simulink model "ES248B_MotAgArbn"  (R2013b)
settings: Solver=FixedStepDiscrete  SolverMode=SingleTasking  StartTime=0.0  StopTime=1  FixedStep=0.0005  RelTol=1e-3
values from neighbouring files (symbols this model uses):
  MAXSTALL_CNT_U08 = DataDict.Constant    [ES248B_MotAgArbn_DataDict.m]
undefined symbols (not defined in the file or in its folder): sigbuilder_block
libraries: simulink x4
settings Model: ModifiedHistory=Rev 008: Updated model to Matlab 2013B, added comments to show requirement linkage  Creator=nz3zln  LastModifiedBy=TZBSJD
settings SolverCC: AutoInsertRateTranBlk=on  InsertRTBMode=Always
settings DataIOCC: LimitDataPoints=off  SaveFormat=Structure  ReturnWorkspaceOutputs=on
settings OptimizationCC: BlockReduction=off  InlineParams=on  ZeroExternalMemoryAtStartup=off  ZeroInternalMemoryAtStartup=off  OptimizeModelRefInitCode=on  LifeSpan=1
settings DebuggingCC: SignalInfNanChecking=error  SignalRangeChecking=warning  UnderspecifiedInitializationDetection=Simplified  SolverPrmCheckMsg=error  InheritedTsInSrcMsg=error  DiscreteInheritContinuousMsg=error  SingleTaskRateTransMsg=error  TasksWithSamePriorityMsg=error  SigSpecEnsureSampleTimeMsg=error  CheckMatrixSingularityMsg=error  ParameterUnderflowMsg=error  ParameterPrecisionLossMsg=error  ParameterTunabilityLossMsg=error  FixptConstUnderflowMsg=warning  FixptConstOverflowMsg=warning  VectorMatrixConversionMsg=error  SignalLabelMismatchMsg=error  UnconnectedInputMsg=error  UnconnectedOutputMsg=error  UnconnectedLineMsg=error  SFcnCompatibilityMsg=error  UniqueDataStoreMsg=warning  BusObjectLabelMismatch=error  RootOutportRequireBusObject=error  AssertControl=DisableAll  ModelReferenceIOMsg=error  ModelReferenceVersionMismatchMessage=warning  ModelReferenceIOMismatchMessage=error  ModelReferenceCSMismatchMessage=warning  ModelReferenceDataLoggingMessage=error  StateNameClashWarn=warning  StrictBusMsg=ErrorOnBusTreatedAsVector  NonBusSignalsTreatedAsBus=error  SFUnexpectedBacktrackingDiag=error  SFInvalidInputDataAccessInChartInitDiag=error  SFNoUnconditionalDefaultTransitionDiag=error  SFTransitionOutsideNaturalParentDiag=error  SFUnconditionalTransitionShadowingDiag=error  SFUndirectedBroadcastEventsDiag=error
settings ModelReferenceCC: ModelReferenceNumInstancesAllowed=Single
settings RTWCC: SystemTargetFile=autosar.tlc  GenCodeOnly=on  TemplateMakefile=ert_default_tmf  Description=AUTOSAR  GenerateReport=on  ProcessScript=autosar_make_rtw_hook  LaunchReport=on
settings CodeAppCC: GenerateComments=off  IgnoreCustomStorageClasses=off  CustomSymbolStrType=$N$R$M  CustomSymbolStrBlkIO=$N$M  SimulinkBlockComments=off
settings STFCustomTargetCC: ParMdlRefBuildCompliant=on  CompOptLevelCompliant=on  IncludeMdlTerminateFcn=off  CombineOutputUpdateFcns=on  SuppressErrorStatus=on  ERTFirstTimeCompliant=on  ERTCustomFileBanners=on  SupportNonFinite=off  SupportComplex=off  SupportContinuousTime=off  SupportNonInlinedSFcns=off  MATLABClassNameForMDSCustomization=Simulink.SoftwareTarget.ERTCustomization  AutosarCompliant=on  GRTInterface=off  SystemTargetFile=autosar.tlc
settings ERTTargetCC: CodeReplacementLibrary=ANSI_C  ConcurrentExecutionCompliant=off  IncludeMdlTerminateFcn=off  SuppressErrorStatus=on  SupportNonFinite=off  SupportComplex=off  ModelStepFunctionPrototypeControlCompliant=off  CPPClassGenCompliant=off  AutosarCompliant=on  InlinedParameterPlacement=NonHierarchical  ERTCustomFileTemplate=example_file_process.tlc  EnableUserReplacementTypes=on

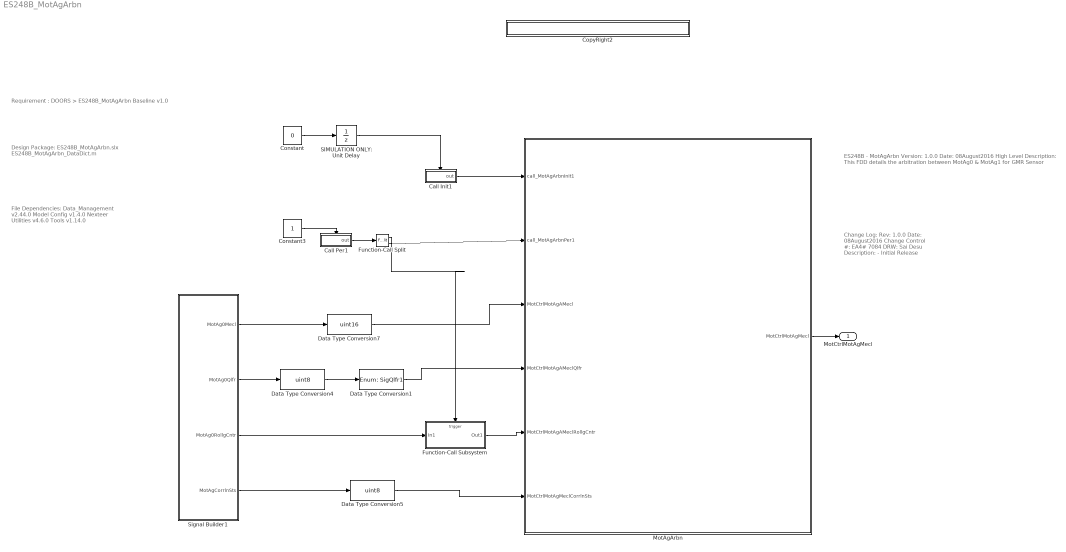
== system ES248B_MotAgArbn ==
  note: ES248B - MotAgArbn
      |
      | Version: 1.0.0
      | Date: 08August2016
      |
      | High Level Description:
      | This FDD details the arbitration between MotAg0 & MotAg1 for GMR Sensor
  note: Change Log:
      |
      | Rev: 1.0.0
      | Date: 08August2016
      | Change Control #: EA4# 7084
      | DRW: Sai Desu
      | Description:
      | - Initial Release
  note: File Dependencies:
      | Data_Management v2.44.0
      | Model Config v1.4.0
      | Nexteer Utilities v4.6.0
      | Tools v1.14.0
  note: Requirement :
      |
      | DOORS > ES248B_MotAgArbn  Baseline  v1.0
  note: Design Package:
      | ES248B_MotAgArbn.slx
      | ES248B_MotAgArbn_DataDict.m
  Call Init1 : Subsystem  TreatAsAtomicUnit=on
  Call Per1 : Subsystem  TreatAsAtomicUnit=on
  Constant : Constant  Value=0  OutDataTypeStr=uint8
  Constant3 : Constant  OutDataTypeStr=int8
  CopyRight2 : Subsystem  Description=|  mask(Copyright Information){none=on}
      | Copyright info block.                                               
      |                                                                     
      | Place copyright information at the top of every subsystem in design.
      mask prompts: none "No parameters"
      mask help: Place copyright information at the top of every subsystem in design.
      mask Display:
      | NxtrConf = 'Nexteer Confidential';
      | 
      | sys = bdroot; %handle for the current model ("system")
      | first = get_param(sys,'Created');
      | first = first(end-3:end);  %year is last four digits
      | 
      | last = get_param(sys,'LastModifiedDate');
      | if isempty(last)
      |     last = datestr(now,'yyyy');
      | else
      |     last = last(end-3:end);
      | end
      | 
      | if strcmp(first,last)
      |     fprintf('%s -- Copyright %s Nexteer',NxtrConf,first)
      | else
      |     fprintf('%s -- %s%s- %s Nexteer',NxtrConf,char(169),first,last)
      | end
  Data Type Conversion1 : DataTypeConversion  OutDataTypeStr=Enum: SigQlfr1
  Data Type Conversion4 : DataTypeConversion  OutDataTypeStr=uint8  RndMeth=Nearest
  Data Type Conversion5 : DataTypeConversion  OutDataTypeStr=uint8  RndMeth=Nearest
  Data Type Conversion7 : DataTypeConversion  OutDataTypeStr=uint16  RndMeth=Nearest
  Function-Call Split : FunctionCallSplit
  Function-Call Subsystem : Subsystem  TreatAsAtomicUnit=on
  MotAgArbn : Subsystem
  SIMULATION ONLY: Unit Delay : UnitDelay  InitialCondition=1  SampleTime=-1
  Signal Builder1 : Subsystem  Tag=STV Subsys  LoadFcn=sigbuilder_block('load');  StartFcn=sigbuilder_block('start');  StopFcn=sigbuilder_block('stop');  ClipboardFcn=sigbuilder_block('clipboard');  mask(Sigbuilder block){}
      mask help: Simulink:masks:SigbuilderBlock_MD
      mask init:
      | if ~strcmp(get_param(bdroot(gcbh),'SimulationStatus'),'stopped') tuvar = sigbuilder_block('maskInit'); end
      settings: CopyFcn=sigbuilder_block('copy');  DeleteFcn=sigbuilder_block('delete');  ModelCloseFcn=sigbuilder_block('modelClose');  PreSaveFcn=sigbuilder_block('preSave');  PauseFcn=sigbuilder_block('pause');  ContinueFcn=sigbuilder_block('continue');  NameChangeFcn=sigbuilder_block('namechange');  OpenFcn=sigbuilder_block('open',[1440 0 1440 753 ]);  CloseFcn=sigbuilder_block('close');
      mask Display: plot(0, 0, 100, 100,[2, 2, 32, 32, 2], [68, 8, 8, 68, 68],[32, 2], [38, 38], [32, 19, 2],[53, 60, 44], [32, 17, 17, 2],[16, 16, 31, 31]);txt = getActiveGroup(gcbh);text(2, 100, txt,'verticalAlignment', 'top');
  MotCtrlMotAgMecl : Outport
  wires:
  Constant3/1 -> Call Per1/Enable
  Call Per1/1(out) -> Function-Call Split/1
  Signal Builder1/4(MotAgCorrlnSts) -> Data Type Conversion5/1
  Signal Builder1/2(MotAg0Qlfr) -> Data Type Conversion4/1
  Signal Builder1/1(MotAg0Mecl) -> Data Type Conversion7/1
  Data Type Conversion4/1 -> Data Type Conversion1/1
  Data Type Conversion5/1 -> MotAgArbn/6(MotCtrlMotAgMeclCorrlnSts)
  Data Type Conversion7/1 -> MotAgArbn/3(MotCtrlMotAgAMecl)
  Function-Call Subsystem/1(Out1) -> MotAgArbn/5(MotCtrlMotAgAMeclRollgCntr)
  Signal Builder1/3(MotAg0RollgCntr) -> Function-Call Subsystem/1(In1)
  Function-Call Split/2 -> MotAgArbn/2(call_MotAgArbnPer1)
  Function-Call Split/1 -> Function-Call Subsystem/Trigger
  Call Init1/1(out) -> MotAgArbn/1(call_MotAgArbnInit1)
  Constant/1 -> SIMULATION ONLY: Unit Delay/1
  SIMULATION ONLY: Unit Delay/1 -> Call Init1/Enable
  MotAgArbn/1(MotCtrlMotAgMecl) -> MotCtrlMotAgMecl/1
  Data Type Conversion1/1 -> MotAgArbn/4(MotCtrlMotAgAMeclQlfr)

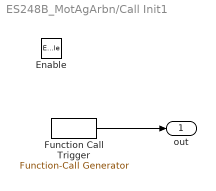
== system ES248B_MotAgArbn/Call Init1 ==
  Enable : EnablePort
  Function Call Trigger : simulink/Ports & Subsystems/Function-Call Generator  RequirementInfo={} %GIDa_03d3be70_2a53_4f3d_90ce_b287f92bdd04  sample_time=0.0005  numberOfIterations=1
  out : Outport
  wires:
  Function Call Trigger/1 -> out/1

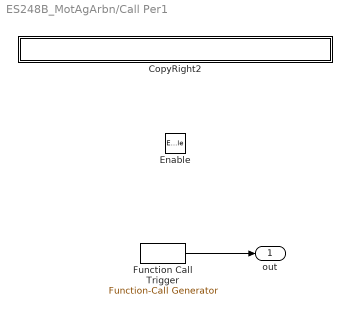
== system ES248B_MotAgArbn/Call Per1 ==
  Enable : EnablePort
  CopyRight2 : Subsystem  Description=|  mask(Copyright Information){none=on}
      | Copyright info block.                                               
      |                                                                     
      | Place copyright information at the top of every subsystem in design.
      mask prompts: none "No parameters"
      mask help: Place copyright information at the top of every subsystem in design.
      mask Display:
      | NxtrConf = 'Nexteer Confidential';
      | 
      | sys = bdroot; %handle for the current model ("system")
      | first = get_param(sys,'Created');
      | first = first(end-3:end);  %year is last four digits
      | 
      | last = get_param(sys,'LastModifiedDate');
      | if isempty(last)
      |     last = datestr(now,'yyyy');
      | else
      |     last = last(end-3:end);
      | end
      | 
      | if strcmp(first,last)
      |     fprintf('%s -- Copyright %s Nexteer',NxtrConf,first)
      | else
      |     fprintf('%s -- %s%s- %s Nexteer',NxtrConf,char(169),first,last)
      | end
  Function Call Trigger : simulink/Ports & Subsystems/Function-Call Generator  RequirementInfo={} %GIDa_6dd05ab1_f91b_4d7a_a0ec_1170d213fa7b  sample_time=0.0005  numberOfIterations=1
  out : Outport
  wires:
  Function Call Trigger/1 -> out/1

== system ES248B_MotAgArbn/CopyRight2 ==

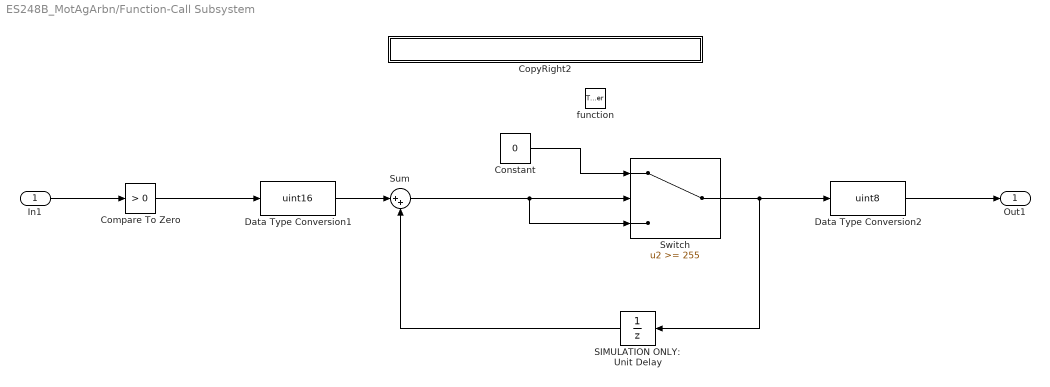
== system ES248B_MotAgArbn/Function-Call Subsystem ==
  In1 : Inport
  function : TriggerPort  TriggerType=function-call
  Compare To Zero : simulink/Logic and Bit Operations/Compare To Zero  relop=>  OutDataTypeStr=uint8
  Constant : Constant  Value=0  OutDataTypeStr=uint16
  CopyRight2 : Subsystem  Description=|  mask(Copyright Information){none=on}
      | Copyright info block.                                               
      |                                                                     
      | Place copyright information at the top of every subsystem in design.
      mask prompts: none "No parameters"
      mask help: Place copyright information at the top of every subsystem in design.
      mask Display:
      | NxtrConf = 'Nexteer Confidential';
      | 
      | sys = bdroot; %handle for the current model ("system")
      | first = get_param(sys,'Created');
      | first = first(end-3:end);  %year is last four digits
      | 
      | last = get_param(sys,'LastModifiedDate');
      | if isempty(last)
      |     last = datestr(now,'yyyy');
      | else
      |     last = last(end-3:end);
      | end
      | 
      | if strcmp(first,last)
      |     fprintf('%s -- Copyright %s Nexteer',NxtrConf,first)
      | else
      |     fprintf('%s -- %s%s- %s Nexteer',NxtrConf,char(169),first,last)
      | end
  Data Type Conversion1 : DataTypeConversion  OutDataTypeStr=uint16  RndMeth=Nearest
  Data Type Conversion2 : DataTypeConversion  OutDataTypeStr=uint8  RndMeth=Nearest
  SIMULATION ONLY: Unit Delay : UnitDelay  SampleTime=-1
  Sum : Sum  Inputs=|++
  Switch : Switch  Threshold=255
  Out1 : Outport
  wires:
  Constant/1 -> Switch/1
  Sum/1 -> Switch/3, Switch/2
  Data Type Conversion1/1 -> Sum/1
  Switch/1 -> SIMULATION ONLY: Unit Delay/1, Data Type Conversion2/1
  Data Type Conversion2/1 -> Out1/1
  SIMULATION ONLY: Unit Delay/1 -> Sum/2
  In1/1 -> Compare To Zero/1
  Compare To Zero/1 -> Data Type Conversion1/1

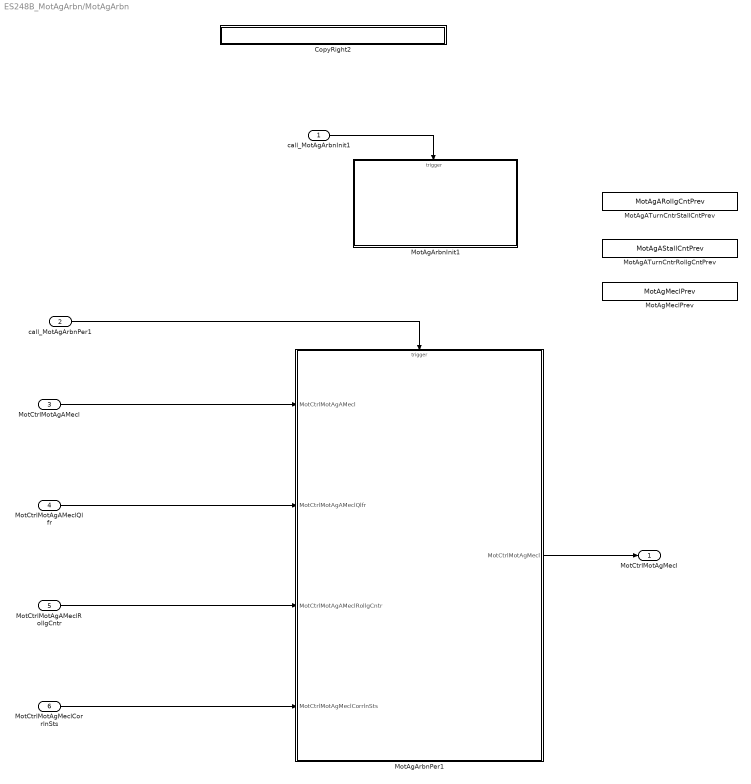
== system ES248B_MotAgArbn/MotAgArbn ==
  call_MotAgArbnInit1 : Inport  RequirementInfo={} %GIDa_2de43c09_82b6_47b9_8e99_1c21e4b82fe2
  call_MotAgArbnPer1 : Inport  RequirementInfo={} %GIDa_468d2479_6710_42ce_bd19_b69834ab6306  Port=2
  MotCtrlMotAgAMecl : Inport  Port=3
  MotCtrlMotAgAMeclQlfr : Inport  Port=4
  MotCtrlMotAgAMeclRollgCntr : Inport  RequirementInfo={} %GIDa_84fb02b3_72b4_4e28_a17f_e99f7297de00  Port=5
  MotCtrlMotAgMeclCorrlnSts : Inport  Port=6
  CopyRight2 : Subsystem  Description=|  mask(Copyright Information){none=on}
      | Copyright info block.                                               
      |                                                                     
      | Place copyright information at the top of every subsystem in design.
      mask prompts: none "No parameters"
      mask help: Place copyright information at the top of every subsystem in design.
      mask Display:
      | NxtrConf = 'Nexteer Confidential';
      | 
      | sys = bdroot; %handle for the current model ("system")
      | first = get_param(sys,'Created');
      | first = first(end-3:end);  %year is last four digits
      | 
      | last = get_param(sys,'LastModifiedDate');
      | if isempty(last)
      |     last = datestr(now,'yyyy');
      | else
      |     last = last(end-3:end);
      | end
      | 
      | if strcmp(first,last)
      |     fprintf('%s -- Copyright %s Nexteer',NxtrConf,first)
      | else
      |     fprintf('%s -- %s%s- %s Nexteer',NxtrConf,char(169),first,last)
      | end
  MotAgATurnCntrRollgCntPrev : DataStoreMemory  DataStoreName=MotAgAStallCntPrev  StateMustResolveToSignalObject=on
  MotAgATurnCntrStallCntPrev : DataStoreMemory  DataStoreName=MotAgARollgCntPrev  StateMustResolveToSignalObject=on
  MotAgArbnInit1 : Subsystem
  MotAgArbnPer1 : Subsystem  TreatAsAtomicUnit=on
  MotAgMeclPrev : DataStoreMemory  DataStoreName=MotAgMeclPrev  StateMustResolveToSignalObject=on
  MotCtrlMotAgMecl : Outport
  wires:
  call_MotAgArbnPer1/1 -> MotAgArbnPer1/Trigger
  MotAgArbnPer1/1(MotCtrlMotAgMecl) -> MotCtrlMotAgMecl/1
  MotCtrlMotAgAMecl/1 -> MotAgArbnPer1/1(MotCtrlMotAgAMecl)
  MotCtrlMotAgAMeclQlfr/1 -> MotAgArbnPer1/2(MotCtrlMotAgAMeclQlfr)
  MotCtrlMotAgMeclCorrlnSts/1 -> MotAgArbnPer1/4(MotCtrlMotAgMeclCorrlnSts)
  call_MotAgArbnInit1/1 -> MotAgArbnInit1/Trigger
  MotCtrlMotAgAMeclRollgCntr/1 -> MotAgArbnPer1/3(MotCtrlMotAgAMeclRollgCntr)

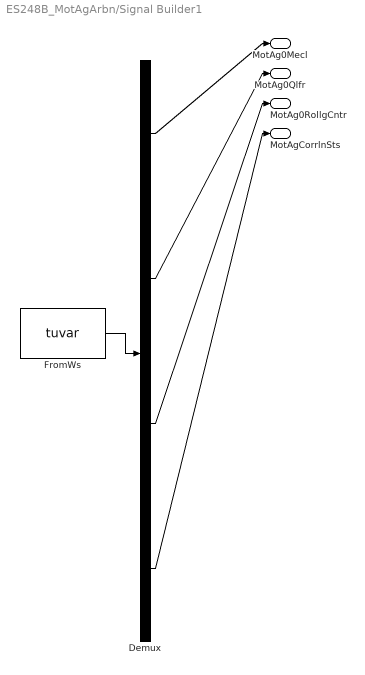
== system ES248B_MotAgArbn/Signal Builder1 ==
  Demux : Demux  Tag=STV Demux
  FromWs : FromWorkspace  Tag=STV FromWs  VariableName=tuvar  SampleTime=0
      SigBuilderData=|
      | common.afterFinalStr = 'Extrapolate'
      | common.sampleTime = 0
      | dataSet(1).timeRange = [0 1]
      | dataSet(1).name = 'Group 1'
      | dataSet(2).timeRange = [0 1]
      | dataSet(2).name = 'looping'
      | dataSet(3).timeRange = [0 1]
      | dataSet(3).name = 'TotalFial'
      | dataSet(4).timeRange = [0 1]
      | dataSet(4).name = 'Allpass'
      | sbobj.Groups(1).Name = 'Group 1'
      | sbobj.Groups(1).Signals(1).Name = 'MotAg0Mecl'
      | sbobj.Groups(1).Signals(1).XData = [0 0.166666666667 0.166666666667 0.333333333333 0.333333333333 0.5 0.5 0.666666666667 0.666666666667 0.833333333333 0.833333333333 0.901 0.901 1]
      | sbobj.Groups(1).Signals(1).YData = [0 65534 0 65534 0 65534 0 65534 0 65534 0 61000 0 60000]
      | sbobj.Groups(1).Signals(2).Name = 'MotAg0Qlfr'
      | sbobj.Groups(1).Signals(2).XData = [0 0.25 0.25 0.4 0.4 0.71 0.71 0.89 0.89 1]
      | sbobj.Groups(1).Signals(2).YData = [1 1 2 2 1 1 2 2 1 1]
      | sbobj.Groups(1).Signals(3).Name = 'MotAg0RollgCntr'
      | sbobj.Groups(1).Signals(3).XData = [0 1]
      | sbobj.Groups(1).Signals(3).YData = [1 1]
      | sbobj.Groups(1).Signals(4).Name = 'MotAgCorrlnSts'
      | sbobj.Groups(1).Signals(4).XData = [0 0.501 0.501 0.599 0.599 0.98 0.98 1]
      | sbobj.Groups(1).Signals(4).YData = [3 3 2 2 3 3 0 2]
      | sbobj.Groups(1).TimeRange = [0 1]
      | sbobj.Groups(2).Name = 'looping'
      | sbobj.Groups(2).Signals(1).Name = 'MotAg0Mecl'
      | sbobj.Groups(2).Signals(1).XData = [0 0.166666666667 0.166666666667 0.333333333333 0.333333333333 0.5 0.5 0.666666666667 0.666666666667 0.833333333333 0.833333333333 0.901 0.901 1]
      | sbobj.Groups(2).Signals(1).YData = [0 65534 0 65534 0 65534 0 65534 0 65534 0 61000 0 60000]
      | sbobj.Groups(2).Signals(2).Name = 'MotAg0Qlfr'
      | sbobj.Groups(2).Signals(2).XData = [0 0.25 0.4 0.71 0.71 0.89 0.89 1]
      | sbobj.Groups(2).Signals(2).YData = [1 1 1 1 2 2 1 1]
      | sbobj.Groups(2).Signals(3).Name = 'MotAg0RollgCntr'
      | sbobj.Groups(2).Signals(3).XData = [0 0.6 0.6 1]
      | sbobj.Groups(2).Signals(3).YData = [0 0 1 1]
      | sbobj.Groups(2).Signals(4).Name = 'MotAgCorrlnSts'
      | sbobj.Groups(2).Signals(4).XData = [0 0.201 0.201 0.3 0.3 0.501 0.599 0.633 0.633 0.667 0.667 0.98 0.98 1]
      | sbobj.Groups(2).Signals(4).YData = [3 3 1 1 3 3 3 3 0 0 3 3 0 2]
      | sbobj.Groups(2).TimeRange = [0 1]
      | sbobj.Groups(3).Name = 'TotalFial'
      | sbobj.Groups(3).Signals(1).Name = 'MotAg0Mecl'
      | sbobj.Groups(3).Signals(1).XData = [0 0.166666666667 0.166666666667 0.333333333333 0.333333333333 0.5 0.5 0.666666666667 0.666666666667 0.833333333333 0.833333333333 0.901 0.901 1]
      | sbobj.Groups(3).Signals(1).YData = [0 65534 0 65534 0 65534 0 65534 0 65534 0 61000 0 60000]
      | sbobj.Groups(3).Signals(2).Name = 'MotAg0Qlfr'
      | sbobj.Groups(3).Signals(2).XData = [0 0.04 0.04 0.1 0.25 0.4 0.7 0.7 0.89 0.89 1]
      | sbobj.Groups(3).Signals(2).YData = [2 2 1 1 1 1 1 2 2 1 1]
      | sbobj.Groups(3).Signals(3).Name = 'MotAg0RollgCntr'
      | sbobj.Groups(3).Signals(3).XData = [0 0.04 0.04 0.6 0.6 0.85 0.85 1]
      | sbobj.Groups(3).Signals(3).YData = [1 1 0 0 1 1 0 0]
      | sbobj.Groups(3).Signals(4).Name = 'MotAgCorrlnSts'
      | sbobj.Groups(3).Signals(4).XData = [0 0.201 0.201 0.3 0.3 0.501 0.599 0.599 0.7 0.7 0.98 0.98 1]
      | sbobj.Groups(3).Signals(4).YData = [3 3 1 1 3 3 3 0 0 3 3 0 2]
      | sbobj.Groups(3).TimeRange = [0 1]
      | sbobj.Groups(4).Name = 'Allpass'
      | sbobj.Groups(4).Signals(1).Name = 'MotAg0Mecl'
      | sbobj.Groups(4).Signals(1).XData = [0 0.166666666667 0.166666666667 0.333333333333 0.333333333333 0.5 0.5 0.666666666667 0.666666666667 0.833333333333 0.833333333333 0.901 0.901 1]
      | sbobj.Groups(4).Signals(1).YData = [0 65534 0 65534 0 65534 0 65534 0 65534 0 61000 0 60000]
      | sbobj.Groups(4).Signals(2).Name = 'MotAg0Qlfr'
      | sbobj.Groups(4).Signals(2).XData = [0 0.25 0.4 0.7 0.89 1]
      | sbobj.Groups(4).Signals(2).YData = [1 1 1 1 1 1]
      | sbobj.Groups(4).Signals(3).Name = 'MotAg0RollgCntr'
      | sbobj.Groups(4).Signals(3).XData = [0 0.6 0.89 1]
      | sbobj.Groups(4).Signals(3).YData = [1 1 1 1]
      | sbobj.Groups(4).Signals(4).Name = 'MotAgCorrlnSts'
      | sbobj.Groups(4).Signals(4).XData = [0 0.201 0.201 0.3 0.3 0.501 0.599 0.599 0.7 0.7 0.98 0.98 1]
      | sbobj.Groups(4).Signals(4).YData = [3 3 1 1 3 3 3 1 1 3 3 1 1]
      | sbobj.Groups(4).TimeRange = [0 1]
  MotAg0Mecl : Outport  Tag=STV Outport
  MotAg0Qlfr : Outport  Tag=STV Outport  Port=2
  MotAg0RollgCntr : Outport  Tag=STV Outport  Port=3
  MotAgCorrlnSts : Outport  Tag=STV Outport  Port=4
  wires:
  FromWs/1 -> Demux/1
  Demux/1 -> MotAg0Mecl/1
  Demux/2 -> MotAg0Qlfr/1
  Demux/3 -> MotAg0RollgCntr/1
  Demux/4 -> MotAgCorrlnSts/1

== system ES248B_MotAgArbn/Call Per1/CopyRight2 ==

== system ES248B_MotAgArbn/Function-Call Subsystem/CopyRight2 ==

== system ES248B_MotAgArbn/MotAgArbn/CopyRight2 ==

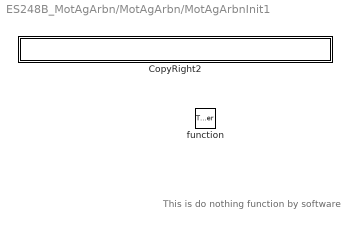
== system ES248B_MotAgArbn/MotAgArbn/MotAgArbnInit1 ==
  note: This is do nothing function by software
  function : TriggerPort  TriggerType=function-call
  CopyRight2 : Subsystem  Description=|  mask(Copyright Information){none=on}
      | Copyright info block.                                               
      |                                                                     
      | Place copyright information at the top of every subsystem in design.
      mask prompts: none "No parameters"
      mask help: Place copyright information at the top of every subsystem in design.
      mask Display:
      | NxtrConf = 'Nexteer Confidential';
      | 
      | sys = bdroot; %handle for the current model ("system")
      | first = get_param(sys,'Created');
      | first = first(end-3:end);  %year is last four digits
      | 
      | last = get_param(sys,'LastModifiedDate');
      | if isempty(last)
      |     last = datestr(now,'yyyy');
      | else
      |     last = last(end-3:end);
      | end
      | 
      | if strcmp(first,last)
      |     fprintf('%s -- Copyright %s Nexteer',NxtrConf,first)
      | else
      |     fprintf('%s -- %s%s- %s Nexteer',NxtrConf,char(169),first,last)
      | end

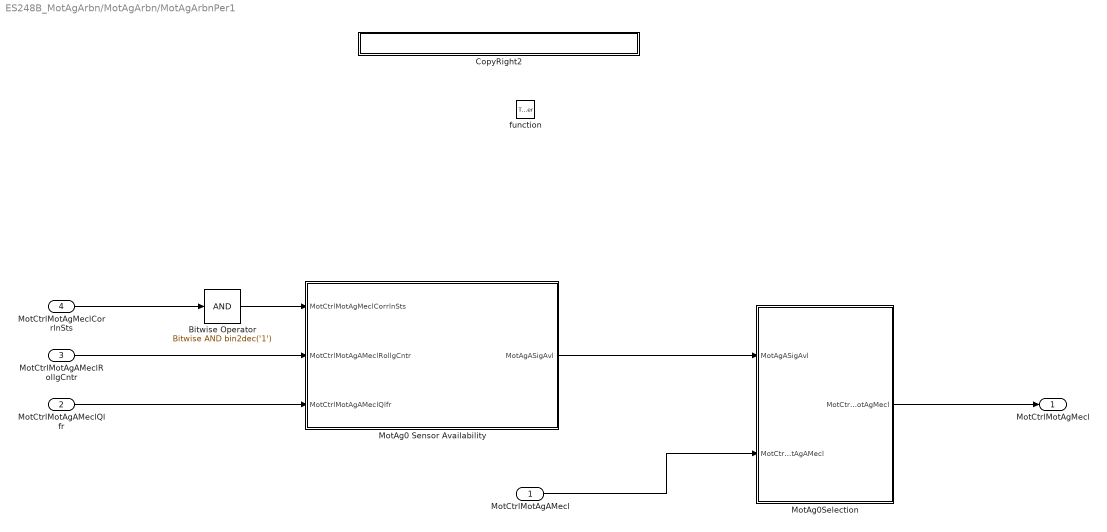
== system ES248B_MotAgArbn/MotAgArbn/MotAgArbnPer1 ==
  MotCtrlMotAgAMecl : Inport
  MotCtrlMotAgAMeclQlfr : Inport  Port=2
  MotCtrlMotAgAMeclRollgCntr : Inport  RequirementInfo={} %GIDa_9d4de4cc_7719_48bf_85c0_912168cfd52f  Port=3
  MotCtrlMotAgMeclCorrlnSts : Inport  Port=4
  function : TriggerPort  TriggerType=function-call
  Bitwise Operator : simulink/Logic and Bit Operations/Bitwise Operator  logicop=AND  UseBitMask=on  BitMask=bin2dec('1')  BitMaskRealWorld=Stored Integer
  CopyRight2 : Subsystem  Description=|  mask(Copyright Information){none=on}
      | Copyright info block.                                               
      |                                                                     
      | Place copyright information at the top of every subsystem in design.
      mask prompts: none "No parameters"
      mask help: Place copyright information at the top of every subsystem in design.
      mask Display:
      | NxtrConf = 'Nexteer Confidential';
      | 
      | sys = bdroot; %handle for the current model ("system")
      | first = get_param(sys,'Created');
      | first = first(end-3:end);  %year is last four digits
      | 
      | last = get_param(sys,'LastModifiedDate');
      | if isempty(last)
      |     last = datestr(now,'yyyy');
      | else
      |     last = last(end-3:end);
      | end
      | 
      | if strcmp(first,last)
      |     fprintf('%s -- Copyright %s Nexteer',NxtrConf,first)
      | else
      |     fprintf('%s -- %s%s- %s Nexteer',NxtrConf,char(169),first,last)
      | end
  MotAg0 Sensor Availability : Subsystem  RequirementInfo={} %GIDa_a3666822_1018_404e_9f7a_19faaace6442  TreatAsAtomicUnit=on
  MotAg0Selection : Subsystem  RequirementInfo={} %GIDa_85a2964f_79da_4020_bfb6_043b97388858
  MotCtrlMotAgMecl : Outport
  wires:
  MotCtrlMotAgMeclCorrlnSts/1 -> Bitwise Operator/1
  Bitwise Operator/1 -> MotAg0 Sensor Availability/1(MotCtrlMotAgMeclCorrlnSts)
  MotCtrlMotAgAMeclQlfr/1 -> MotAg0 Sensor Availability/3(MotCtrlMotAgAMeclQlfr)
  MotAg0 Sensor Availability/1(MotAgASigAvl) -> MotAg0Selection/1(MotAgASigAvl)
  MotCtrlMotAgAMecl/1 -> MotAg0Selection/2(MotCtrlMotAgAMecl)
  MotCtrlMotAgAMeclRollgCntr/1 -> MotAg0 Sensor Availability/2(MotCtrlMotAgAMeclRollgCntr)
  MotAg0Selection/1("MotCtrlMotAgMecl ") -> MotCtrlMotAgMecl/1

== system ES248B_MotAgArbn/MotAgArbn/MotAgArbnInit1/CopyRight2 ==

== system ES248B_MotAgArbn/MotAgArbn/MotAgArbnPer1/CopyRight2 ==

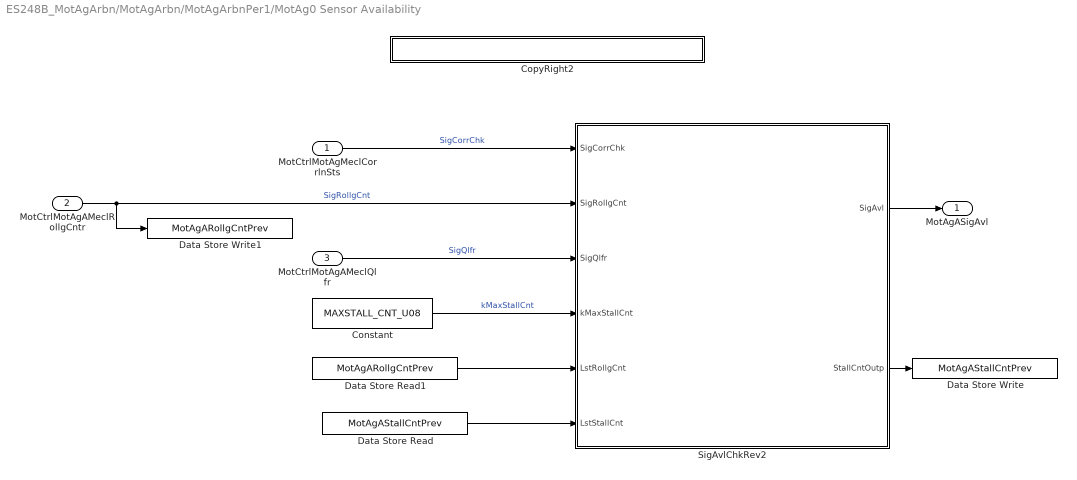
== system ES248B_MotAgArbn/MotAgArbn/MotAgArbnPer1/MotAg0 Sensor Availability ==
  MotCtrlMotAgMeclCorrlnSts : Inport
  MotCtrlMotAgAMeclRollgCntr : Inport  Port=2
  MotCtrlMotAgAMeclQlfr : Inport  Port=3
  Constant : Constant  Value=MAXSTALL_CNT_U08
  CopyRight2 : Subsystem  Description=|  mask(Copyright Information){none=on}
      | Copyright info block.                                               
      |                                                                     
      | Place copyright information at the top of every subsystem in design.
      mask prompts: none "No parameters"
      mask help: Place copyright information at the top of every subsystem in design.
      mask Display:
      | NxtrConf = 'Nexteer Confidential';
      | 
      | sys = bdroot; %handle for the current model ("system")
      | first = get_param(sys,'Created');
      | first = first(end-3:end);  %year is last four digits
      | 
      | last = get_param(sys,'LastModifiedDate');
      | if isempty(last)
      |     last = datestr(now,'yyyy');
      | else
      |     last = last(end-3:end);
      | end
      | 
      | if strcmp(first,last)
      |     fprintf('%s -- Copyright %s Nexteer',NxtrConf,first)
      | else
      |     fprintf('%s -- %s%s- %s Nexteer',NxtrConf,char(169),first,last)
      | end
  Data Store Read : DataStoreRead  DataStoreName=MotAgAStallCntPrev
  Data Store Read1 : DataStoreRead  DataStoreName=MotAgARollgCntPrev
  Data Store Write : DataStoreWrite  RequirementInfo={} %GIDa_9a9cd5ba_32cc_4b15_9fbb_ffc99f86186c  DataStoreName=MotAgAStallCntPrev
  Data Store Write1 : DataStoreWrite  RequirementInfo={} %GIDa_68fbb913_cad7_4656_a0fb_1b4163fceb61  DataStoreName=MotAgARollgCntPrev
  SigAvlChkRev2 : Stateflow chart  RequirementInfo="{'linktype_rmi_doors' '00011b4a (/ESG Group/FDD Module Requirements/EA4 Specific/ES248B_MotAgArbn)' '#ES248B_35' 'true' 'REQ:  ES248B_35' '' } %GIDa_ec1912f1_c7f6_4114_866c_684914a13f21"  TreatAsAtomicUnit=on
  MotAgASigAvl : Outport  RequirementInfo="{'linktype_rmi_doors' '00011b4a (/ESG Group/FDD Module Requirements/EA4 Specific/ES248B_MotAgArbn)' '#ES248B_35' 'true' 'REQ:  ES248B_35' '' } %GIDa_8d8daaab_601a_421a_88d3_d4e0374f5eae"
  wires:
  MotCtrlMotAgMeclCorrlnSts/1 -> SigAvlChkRev2/1(SigCorrChk)  "SigCorrChk"
  MotCtrlMotAgAMeclRollgCntr/1 -> Data Store Write1/1, SigAvlChkRev2/2(SigRollgCnt)  "SigRollgCnt"
  MotCtrlMotAgAMeclQlfr/1 -> SigAvlChkRev2/3(SigQlfr)  "SigQlfr"
  Constant/1 -> SigAvlChkRev2/4(kMaxStallCnt)  "kMaxStallCnt"
  SigAvlChkRev2/1(SigAvl) -> MotAgASigAvl/1
  Data Store Read1/1 -> SigAvlChkRev2/5(LstRollgCnt)
  Data Store Read/1 -> SigAvlChkRev2/6(LstStallCnt)
  SigAvlChkRev2/2(StallCntOutp) -> Data Store Write/1

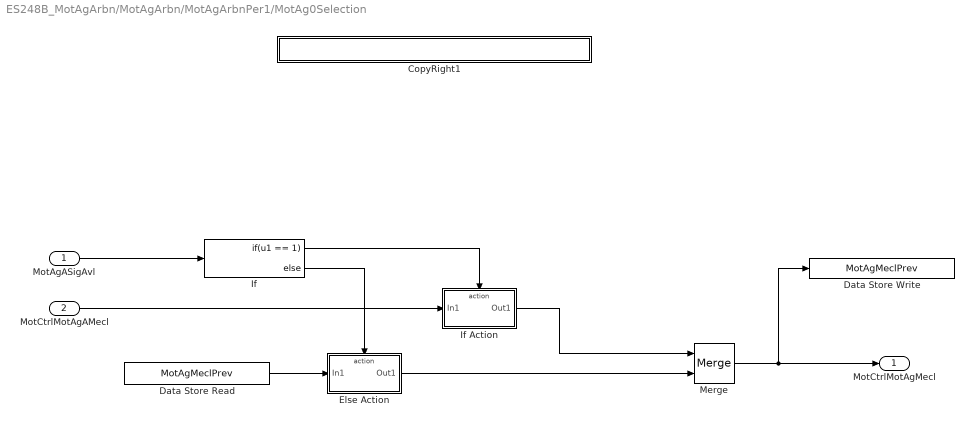
== system ES248B_MotAgArbn/MotAgArbn/MotAgArbnPer1/MotAg0Selection ==
  MotAgASigAvl : Inport  RequirementInfo={} %GIDa_deb1ac0e_3c1d_4ef0_9af7_3d519e5bcd6e
  MotCtrlMotAgAMecl : Inport  RequirementInfo={} %GIDa_7a93900a_c68c_4a42_989e_cc2bfe8ec6f3  Port=2
  CopyRight1 : Subsystem  Description=|  mask(Copyright Information){none=on}
      | Copyright info block.                                               
      |                                                                     
      | Place copyright information at the top of every subsystem in design.
      mask prompts: none "No parameters"
      mask help: Place copyright information at the top of every subsystem in design.
      mask Display:
      | NxtrConf = 'Nexteer Confidential';
      | 
      | sys = bdroot; %handle for the current model ("system")
      | first = get_param(sys,'Created');
      | first = first(end-3:end);  %year is last four digits
      | 
      | last = get_param(sys,'LastModifiedDate');
      | if isempty(last)
      |     last = datestr(now,'yyyy');
      | else
      |     last = last(end-3:end);
      | end
      | 
      | if strcmp(first,last)
      |     fprintf('%s -- Copyright %s Nexteer',NxtrConf,first)
      | else
      |     fprintf('%s -- %s%s- %s Nexteer',NxtrConf,char(169),first,last)
      | end
  Data Store Read : DataStoreRead  DataStoreName=MotAgMeclPrev
  Data Store Write : DataStoreWrite  RequirementInfo={} %GIDa_69657b82_594f_4d82_ad33_b7847062ba4e  DataStoreName=MotAgMeclPrev
  "Else Action " : Subsystem  RequirementInfo="{'linktype_rmi_doors' '00011b4a (/ESG Group/FDD Module Requirements/EA4 Specific/ES248B_MotAgArbn)' '#ES248B_69' 'true' 'REQ:  ES248B_69' '' } %GIDa_d389c035_6a74_4fc2_9fd7_cdbd76bc82db"  TreatAsAtomicUnit=on
  If : If  RequirementInfo={} %GIDa_0161bf22_f7da_4375_a8bb_f7e6e3eaf1fa  IfExpression=u1 == 1
  "If Action " : Subsystem  RequirementInfo="{'linktype_rmi_doors' '00011b4a (/ESG Group/FDD Module Requirements/EA4 Specific/ES248B_MotAgArbn)' '#ES248B_68' 'true' 'REQ:  ES248B_68' '' } %GIDa_e824bcae_7ba6_4238_be9d_ff4993e301b9"  TreatAsAtomicUnit=on
  Merge : Merge  RequirementInfo={} %GIDa_9b6f3e27_799c_4f03_8f54_6f0edc926d56
  "MotCtrlMotAgMecl " : Outport  RequirementInfo="{'linktype_rmi_doors' '00011b4a (/ESG Group/FDD Module Requirements/EA4 Specific/ES248B_MotAgArbn)' '#ES248B_68' 'true' 'REQ:  ES248B_68' '' ; 'linktype_rmi_doors' '00011b4a (/ESG Group/FDD Module Requirements/EA4 Specific/ES248B_MotAgArbn)' '#ES248B_69' 'true' 'REQ:  ES248B_69' '' } %GIDa_baf725e2_0276_4e42_b62c_b1d736b2a824"
  wires:
  MotAgASigAvl/1 -> If/1
  If/1 -> "If Action "/Action
  MotCtrlMotAgAMecl/1 -> "If Action "/1(In1)
  If/2 -> "Else Action "/Action
  "If Action "/1(Out1) -> Merge/1
  Merge/1 -> Data Store Write/1, "MotCtrlMotAgMecl "/1
  "Else Action "/1(Out1) -> Merge/2
  Data Store Read/1 -> "Else Action "/1(In1)

== system ES248B_MotAgArbn/MotAgArbn/MotAgArbnPer1/MotAg0 Sensor Availability/CopyRight2 ==

== system ES248B_MotAgArbn/MotAgArbn/MotAgArbnPer1/MotAg0Selection/CopyRight1 ==

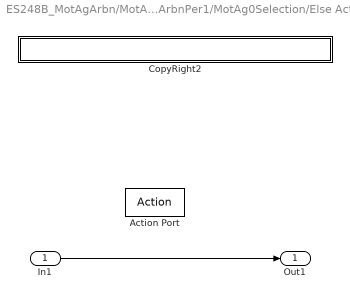
== system ES248B_MotAgArbn/MotAgArbn/MotAgArbnPer1/MotAg0Selection/Else Action  ==
  In1 : Inport
  Action Port : ActionPort  ActionType=else
  CopyRight2 : Subsystem  Description=|  mask(Copyright Information){none=on}
      | Copyright info block.                                               
      |                                                                     
      | Place copyright information at the top of every subsystem in design.
      mask prompts: none "No parameters"
      mask help: Place copyright information at the top of every subsystem in design.
      mask Display:
      | NxtrConf = 'Nexteer Confidential';
      | 
      | sys = bdroot; %handle for the current model ("system")
      | first = get_param(sys,'Created');
      | first = first(end-3:end);  %year is last four digits
      | 
      | last = get_param(sys,'LastModifiedDate');
      | if isempty(last)
      |     last = datestr(now,'yyyy');
      | else
      |     last = last(end-3:end);
      | end
      | 
      | if strcmp(first,last)
      |     fprintf('%s -- Copyright %s Nexteer',NxtrConf,first)
      | else
      |     fprintf('%s -- %s%s- %s Nexteer',NxtrConf,char(169),first,last)
      | end
  Out1 : Outport
  wires:
  In1/1 -> Out1/1

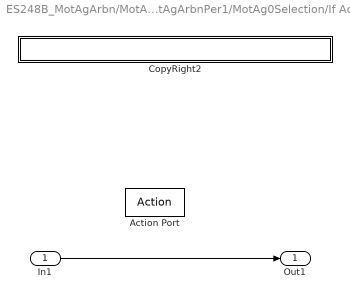
== system ES248B_MotAgArbn/MotAgArbn/MotAgArbnPer1/MotAg0Selection/If Action  ==
  In1 : Inport
  Action Port : ActionPort  ActionType=then
  CopyRight2 : Subsystem  Description=|  mask(Copyright Information){none=on}
      | Copyright info block.                                               
      |                                                                     
      | Place copyright information at the top of every subsystem in design.
      mask prompts: none "No parameters"
      mask help: Place copyright information at the top of every subsystem in design.
      mask Display:
      | NxtrConf = 'Nexteer Confidential';
      | 
      | sys = bdroot; %handle for the current model ("system")
      | first = get_param(sys,'Created');
      | first = first(end-3:end);  %year is last four digits
      | 
      | last = get_param(sys,'LastModifiedDate');
      | if isempty(last)
      |     last = datestr(now,'yyyy');
      | else
      |     last = last(end-3:end);
      | end
      | 
      | if strcmp(first,last)
      |     fprintf('%s -- Copyright %s Nexteer',NxtrConf,first)
      | else
      |     fprintf('%s -- %s%s- %s Nexteer',NxtrConf,char(169),first,last)
      | end
  Out1 : Outport
  wires:
  In1/1 -> Out1/1

== system ES248B_MotAgArbn/MotAgArbn/MotAgArbnPer1/MotAg0Selection/Else Action /CopyRight2 ==

== system ES248B_MotAgArbn/MotAgArbn/MotAgArbnPer1/MotAg0Selection/If Action /CopyRight2 ==

== stateflow chart ES248B_MotAgArbn/MotAgArbn/MotAgArbnPer1/MotAg0 Sensor Availability/SigAvlChkRev2 ==
  note: SigAvl
      | False = 0
      | Pass = 1
  note: SigQlfr
      | 0 = No Result
      | 1 = Pass
      | 2 = Fail
  (default) -> (junction 2)
  (junction 2) -> (junction 4) [order 1] : [SigRollgCnt ==LstRollgCnt]
  (junction 4) -> (junction 7) [order 2] : {
      | StallCntOutp = LstStallCnt +1;
      | }
  (junction 2) -> (junction 3) [order 2]
  (junction 4) -> (junction 7) [order 1] : [LstStallCnt == 255]
      | {
      | StallCntOutp = 255;
      | }
  (junction 3) -> (junction 7) : {
      | StallCntOutp = 0;
      | }
  (junction 7) -> (junction 10)
  (junction 10) -> (junction 12) [order 1] : [StallCntOutp >=kMaxStallCnt]
  (junction 10) -> (junction 14) [order 2]
  (junction 12) -> (junction 17)
  (junction 14) -> (junction 17) [order 2]
  (junction 14) -> (junction 16) [order 1] : [SigQlfr<2 && SigCorrChk>0]
  (junction 17) -> (junction 29) : {
      | SigAvl =0;
      | }
  (junction 16) -> (junction 29) : {
      | SigAvl = 1;
      | }
  data: SigCorrChk input; SigRollgCnt input; SigQlfr input; kMaxStallCnt input; SigAvl output boolean; LstRollgCnt input; LstStallCnt input; StallCntOutp output
